simulink model "BPSK_RC"  (R2020a)
settings: Solver=VariableStepAuto  StartTime=0.0  StopTime=0.1  RelTol=1e-3
values from neighbouring files (symbols this model uses):
  Ac = 1    [init_vars.m]
  alfa = 0.5    [parte2.m]
  fc = 10e3    (= 10000)    [init_vars.m]
  fs = spb*rb    (= 100000)    [init_vars.m]
  rb = 1e3    (= 1000)    [init_vars.m]
  rng_seed = 5    [init_vars.m]
  spb = 100    [init_vars.m]
libraries: commrandsrc3 x1, dspsigops x1, commutil2 x1, commfilt2 x1
settings Model: Creator=pedro  LastModifiedBy=pedro

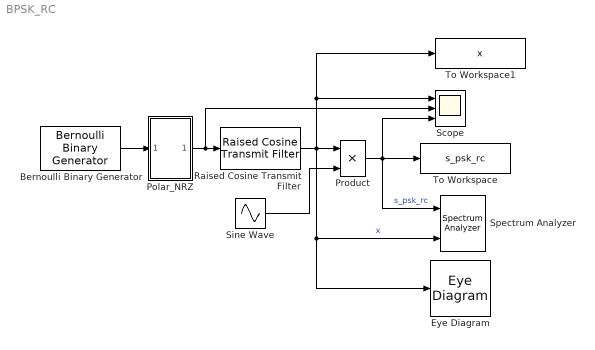
== system BPSK_RC ==
  Bernoulli Binary Generator : commrandsrc3/Bernoulli Binary Generator  ProbabilityOfZero=0.5  SeedSource=Parameter  Seed=rng_seed  SampleTime=1/rb  SamplesPerFrame=1  OutputDataType=double  SimulateUsing=Interpreted execution
  Eye Diagram : EyeDiagram
  Polar_NRZ : Subsystem  mask(Polar_nrz){Rb=rb, Spb=2}
      mask prompts: Rb "Binary Data Rate"; Spb "Samples per bit"
  Product : Product
  Raised Cosine Transmit Filter : commfilt2/Raised Cosine Transmit Filter  filtType=Normal  R=alfa  filtSpan=2  N=spb/2  filterGain=6  InputProcessing=Columns as channels (frame based)  RateOptions=Allow multirate processing  framing=Mute  checkCoeff=off  variableName=rcTxFilt1  checkGain=Normalized  sampMode=Mute  saveAsFlag=0  currentFiltSpan=2  D=(2)/2  launchFVT=on  roundingMode=Floor  overflowMode=off  coeffDataTypeStr=Inherit: Same word length as input  coeffMin=[]  coeffMax=[]  coeffLastDataTypeStr=Inherit: Same word length as input  outputDataTypeStr=Inherit: Same as accumulator  outputMin=[]  outputMax=[]  outputLastDataTypeStr=Inherit: Same as accumulator
  Scope : Scope  NumInputPorts=3
  Sine Wave : Sin  Amplitude=Ac  Frequency=2*pi*fc  SampleTime=1/fs
  Spectrum Analyzer : SpectrumAnalyzer  NumInputPorts=2
  To Workspace : ToWorkspace  VariableName=s_psk_rc  SaveFormat=Timeseries  SampleTime=-1
  To Workspace1 : ToWorkspace  VariableName=x  SaveFormat=Timeseries  SampleTime=-1
  wires:
  Sine Wave/1 -> Product/2
  Bernoulli Binary Generator/1 -> Polar_NRZ/1(In1)
  Product/1 -> Spectrum Analyzer/1, Scope/3, To Workspace/1  "s_psk_rc"
  Polar_NRZ/1(Out1) -> Scope/2, Raised Cosine Transmit Filter/1
  Raised Cosine Transmit Filter/1 -> Product/1, Eye Diagram/1, Spectrum Analyzer/2, To Workspace1/1, Scope/1  "x"

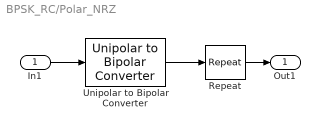
== system BPSK_RC/Polar_NRZ ==
  In1 : Inport
  Repeat : dspsigops/Repeat  N=Spb  InputProcessing=Columns as channels (frame based)  RateOptions=Allow multirate processing  ic=0  mode=Unused parameter value
  Unipolar to Bipolar Converter : commutil2/Unipolar to Bipolar Converter  M=2  polarity=Positive  dataType=Same as input
  Out1 : Outport
  wires:
  Unipolar to Bipolar Converter/1 -> Repeat/1
  In1/1 -> Unipolar to Bipolar Converter/1
  Repeat/1 -> Out1/1
